simulink model "erben_1_ursp_1"  (Simulink 7.8)
settings: Solver=ode45  StartTime=0.0  StopTime=10.0  RelTol=1e-3
values from neighbouring files (symbols this model uses):
  Ts = 1/fs    (= 6.25e-05)    [G722_1.m]    (also in adaptiv_2.m = 0.001; adaptiv_3.m = 0.001; adaptiv_4.m = 0.001; adaptiv_5.m = 0.001)
undefined symbols (not defined in the file or in its folder): ampl
libraries: simulink x1
settings Model: Creator=josef  LastModifiedBy=josef

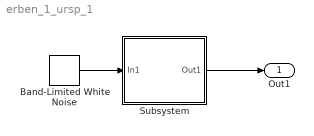
== system erben_1_ursp_1 ==
  Band-Limited White Noise : simulink/Sources/Band-Limited White Noise  Cov=[Ts]  Ts=Ts  seed=[23341]
  Subsystem : Subsystem
  Out1 : Outport
  wires:
  Band-Limited White Noise/1 -> Subsystem/1(In1)
  Subsystem/1(Out1) -> Out1/1

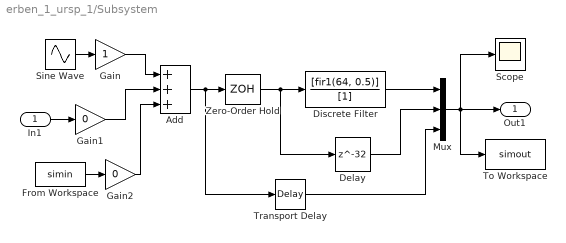
== system erben_1_ursp_1/Subsystem ==
  In1 : Inport
  Add : Sum  Inputs=+++
  Delay : Delay  DelayLength=32
  Discrete Filter : DiscreteFilter  Numerator=[fir1(64, 0.5)]  Denominator=[1]
  From Workspace : FromWorkspace  VariableName=simin  SampleTime=0
  Gain : Gain
  Gain1 : Gain  Gain=0
  Gain2 : Gain  Gain=0
  Mux : Mux  Inputs=3
  Scope : Scope
  Sine Wave : Sin  Amplitude=ampl  Frequency=200*2*pi  SampleTime=0
  To Workspace : ToWorkspace  VariableName=simout  SampleTime=-1  SaveFormat=Structure With Time
  Transport Delay : TransportDelay  DelayTime=Ts*32
  Zero-Order Hold : ZeroOrderHold  SampleTime=Ts
  Out1 : Outport
  wires:
  Add/1 -> Zero-Order Hold/1, Transport Delay/1
  Zero-Order Hold/1 -> Discrete Filter/1, Delay/1
  Discrete Filter/1 -> Mux/1
  Delay/1 -> Mux/2
  Transport Delay/1 -> Mux/3
  Mux/1 -> Scope/1, To Workspace/1, Out1/1
  Sine Wave/1 -> Gain/1
  From Workspace/1 -> Gain2/1
  Gain/1 -> Add/1
  Gain1/1 -> Add/2
  In1/1 -> Gain1/1
  Gain2/1 -> Add/3
